simulink model "fangbo_pll_eso_J_identification"  (R2018b)
settings: Solver=FixedStepAuto  StartTime=0.0  StopTime=0.2  FixedStep=1e-7  RelTol=1e-3
InitFcn:
  | Vin1=30;%注入高频信号幅值
  | fin1=5000;%注入高频信号频率
  | fpwm=10000;%电流环控制频率
  | Tpwm=1/fpwm;
  | Tspd=Tpwm*10;%速度环控制周期（未用）
  | Td=2e-6;%逆变器死区时间（未加入）
  | Udc=90;
  | Pn=4;%极对数
  | R=0.281;
  | Ld=2.523e-3;Lq=5e-3;
  | faif=0.13455;
  | J=0.0012145+ 0.00126+0.0002601;%两个电机加联轴器
  | B=0.0006;
  | TL=10;%额定负载
  | nref=2200;%给定转速
  | %%%%%%luenberger观测器参数%%%%%%%
  | p=2*pi*10;%2;%极点位置，可调
  | eta=1;%1e-2;
  | alpha1=3*p;
  | alpha2=3*p^2;
  | alpha3=p^3;
  | %%%%%%锁相环参数%%%%%%%%%%%%%%%%%
  | Kppll= 300;   %2*p
  | Kipll= 1000;  %p^2
  | %%%%%%%%%双闭环3对PI参数%%%%%%%%%
  | BWc=300*2*pi;%电流环带宽
  | h=6;%速度环中频宽
  | K1=9.55*1.5*Pn*faif/J;
  | wcon=200*2*pi;%转速环反馈滤波和给定滤波器截止频率
  | Tsn=1/BWc+1/wcon;
  | Kpd=BWc*Ld;
  | Kid=R/Ld;
  | Kpq=BWc*Lq;
  | Kiq=R/Lq;
  | Kps=(h+1)/(2*h*Tsn*K1);
  | Kis=1/(h*Tsn);
  | %BWs=15*2*pi;
  | %Kps=BWs/K1;
  | %Kis=Kps*BWs/5;
  | %%%%%%%%%%%扰动观测器PID参数%%%%%%%%%%%%%
  | pd=2*pi*50;
  | kd_d=3*pd;
  | kp_d=3*pd^2;
  | ki_d=pd^3;
undefined symbols (not defined in the file): DiscIntNeverNeededParam, fin
libraries: simulink x16, dsparch4 x7, powerlib x5, dspsrcs4 x2, powerlib_meascontrol x2
(part 1 of 2)
settings Model: Creator=TAH  LastModifiedBy=Think
settings DebuggingCC: LibraryContextMissingDiagnostic=none
settings SFSimCC: SimUseLocalCustomCode=off
settings RTWCC: RTWUseLocalCustomCode=off
settings CodeAppCC: StateflowObjectComments=on
settings SimscapeCC: SimscapeNormalizeSystem=off

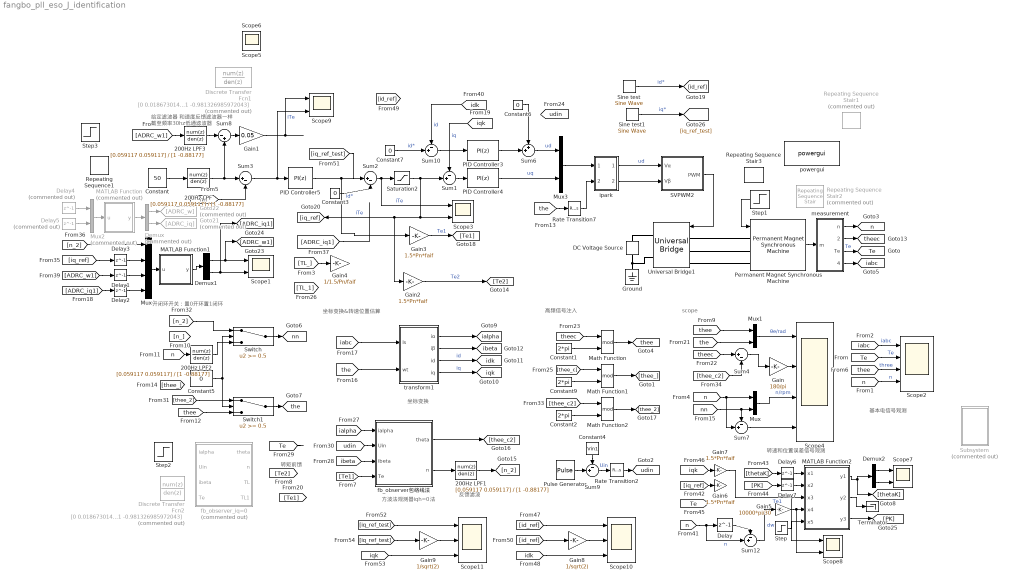
== system fangbo_pll_eso_J_identification ==
  note: 基本电信号观测
  note: 转速和位置误差信号观测
  note: 坐标变换
  note: 给定滤波器
      | 和速度反馈滤波器一样
      | 截至频率30hz低通滤波器
  note: 开闭环开关：置0开环置1闭环
  note: 坐标变换&转速位置估算
  note: 高频信号注入
  note: scope
  note: 方波法观测器iqh=0法
  note: 转矩前馈
  note: 反馈滤波
  200Hz LPF{,1..3} (4 alike) : DiscreteTransferFcn  Numerator=[0.059117 0.059117]  Denominator=[1 -0.88177]  SampleTime=Tpwm
  Constant : Constant  Value=50
  Constant1 : Constant  Value=2*pi  SampleTime=Tpwm
  Constant2 : Constant  Value=2*pi  SampleTime=Tpwm
  Constant3 : Constant  Value=0  SampleTime=1e-4
  Constant4 : Constant  Value=Vin1
  Constant5 : Constant  Value=0
  Constant6 : Constant  Value=0  SampleTime=1e-4
  Constant7 : Constant  Value=0  SampleTime=1e-4
  Constant9 : Constant  Value=2*pi  SampleTime=Tpwm
  DC Voltage Source : powerlib/Electrical Sources/DC Voltage Source  Amplitude=Udc  Measurements=None
      settings: SourceProductName=Simscape Electrical
  Delay{,1..3,6..7} (6 alike) : Delay  DelayLength=1  InitialCondition=0  UseCircularBuffer=on
  Delay4 : Delay  Commented=on  DelayLength=1  InitialCondition=0  UseCircularBuffer=on
  Delay5 : Delay  Commented=on  DelayLength=1  InitialCondition=0  UseCircularBuffer=on
  Demux : Demux  Commented=on  Outputs=2
  Demux1 : Demux  Outputs=2
  Demux2 : Demux  Outputs=2
  Discrete Transfer Fcn1 : DiscreteTransferFcn  Commented=on  Numerator=[0 0.018673014027957]  Denominator=[1 -0.981326985972043]  SampleTime=Tpwm
  Discrete Transfer Fcn2 : DiscreteTransferFcn  Commented=on  Numerator=[0 0.018673014027957]  Denominator=[1 -0.981326985972043]  SampleTime=Tpwm
  Gain : Gain  Gain=180/pi
  Gain1 : Gain  Gain=0.05
  Gain{2..3,6..7} (4 alike) : Gain  Gain=1.5*Pn*faif
  Gain4 : Gain  Gain=1/1.5/Pn/faif
  Gain5 : Gain  Gain=10000*pi/30
  Gain8 : Gain  Gain=1/sqrt(2)
  Gain9 : Gain  Gain=1/sqrt(2)
  Goto21 : Goto  Commented=on  GotoTag=ADRC_iq
  Goto22 : Goto  Commented=on  GotoTag=ADRC_w
  Ground : powerlib/Elements/Ground  LConnTagsString=a
      settings: SourceProductName=Simscape Electrical
  MATLAB Function : MATLAB Function  Commented=on  TreatAsAtomicUnit=on
  MATLAB Function1 : MATLAB Function  TreatAsAtomicUnit=on
  MATLAB Function2 : MATLAB Function  TreatAsAtomicUnit=on
  Math Function : Math  Operator=mod  SaturateOnIntegerOverflow=on
  Math Function1 : Math  Operator=mod  SaturateOnIntegerOverflow=on
  Math Function2 : Math  Operator=mod  SaturateOnIntegerOverflow=on
  Mux : Mux  Inputs=2
  Mux1 : Mux  Inputs=2
  Mux2 : Mux  Commented=on  Inputs=2
  Mux3 : Mux  Inputs=2
  Mux4 : Mux
  PID Controller3 : simulink/Continuous/PID Controller  Controller=PI  Form=Ideal  TimeDomain=Discrete-time  SampleTime=Tpwm  IntegratorMethod=Forward Euler  FilterMethod=Forward Euler  ControllerParametersSource=internal  P=Kpd  I=Kid  D=0  UseFilter=on  N=100  TunerSelectOption=Transfer Function Based (PID Tuner App)  InitialConditionSource=internal  InitialConditionForIntegrator=0  InitialConditionForFilter=0  DifferentiatorICPrevScaledInput=0  ExternalReset=none  TrackingMode=off  Kt=1  LimitOutput=on  UpperSaturationLimit=Udc/sqrt(3)  LowerSaturationLimit=-Udc/sqrt(3)  LinearizeAsGain=on  AntiWindupMode=none  Kb=1  POutMin=[]  POutMax=[]  IOutMin=[]  IOutMax=[]  DOutMin=[]  DOutMax=[]  NOutMin=[]  NOutMax=[]  SumOutMin=[]  SumOutMax=[]  SaturationOutMin=[]  SaturationOutMax=[]  PParamMin=[]  PParamMax=[]  IParamMin=[]  IParamMax=[]  DParamMin=[]  DParamMax=[]  NParamMin=[]  NParamMax=[]  KbParamMin=[]  KbParamMax=[]  KtParamMin=[]  KtParamMax=[]  KbOutMin=[]  KbOutMax=[]  KtOutMin=[]  KtOutMax=[]  IntegratorOutMin=[]  IntegratorOutMax=[]  FilterOutMin=[]  FilterOutMax=[]  SumI1OutMin=[]  SumI1OutMax=[]  SumI2OutMin=[]  SumI2OutMax=[]  SumI3OutMin=[]  SumI3OutMax=[]  SumI4OutMin=[]  SumI4OutMax=[]  SumDOutMin=[]  SumDOutMax=[]  DifferentiatorOutMin=[]  DifferentiatorOutMax=[]  FilterDiffOutCoefMin=[]  FilterDiffOutCoefMax=[]  ReciprocalOutMin=[]  ReciprocalOutMax=[]  SumDenOutMin=[]  SumDenOutMax=[]  SumNumOutMin=[]  SumNumOutMax=[]  DivideOutMin=[]  DivideOutMax=[]  IntegratorContinuousStateAttributes=''  IntegratorStateMustResolveToSignalObject=off  IntegratorRTWStateStorageClass=Auto  FilterContinuousStateAttributes=''  FilterStateMustResolveToSignalObject=off  FilterRTWStateStorageClass=Auto  ParallelPVariant=Passthrough  IdealPVariant=InternalParameters  IVariant=InternalParameters  DVariant=Disabled  IntegratorVariant=Discrete  SatVariant=Enabled  AWVariant=Passthrough  PCopyVariant=Disabled  TRVariant=Disabled  FdbkBlocksVariant=Forward  IdealPFdbkVariant=Disabled  SatFdbkVariant=Disabled  DerivativeFilterVariant=Disabled  NVariant=Disabled  NCopyVariant=Disabled_SignalSpec  FilterICVariant=Disabled  IntegratorICVariant=InternalICs  ExternalResetVariant=Disabled  TRSumVariant=Passthrough  SumFdbkVariant=Disabled  SumVariant=Sum_PI
  PID Controller4 : simulink/Continuous/PID Controller  Controller=PI  Form=Ideal  TimeDomain=Discrete-time  SampleTime=Tpwm  IntegratorMethod=Forward Euler  FilterMethod=Forward Euler  ControllerParametersSource=internal  P=Kpq  I=Kiq  D=0  UseFilter=on  N=100  TunerSelectOption=Transfer Function Based (PID Tuner App)  InitialConditionSource=internal  InitialConditionForIntegrator=0  InitialConditionForFilter=0  DifferentiatorICPrevScaledInput=0  ExternalReset=none  TrackingMode=off  Kt=1  LimitOutput=on  UpperSaturationLimit=Udc/sqrt(3)  LowerSaturationLimit=-Udc/sqrt(3)  LinearizeAsGain=on  AntiWindupMode=none  Kb=1  POutMin=[]  POutMax=[]  IOutMin=[]  IOutMax=[]  DOutMin=[]  DOutMax=[]  NOutMin=[]  NOutMax=[]  SumOutMin=[]  SumOutMax=[]  SaturationOutMin=[]  SaturationOutMax=[]  PParamMin=[]  PParamMax=[]  IParamMin=[]  IParamMax=[]  DParamMin=[]  DParamMax=[]  NParamMin=[]  NParamMax=[]  KbParamMin=[]  KbParamMax=[]  KtParamMin=[]  KtParamMax=[]  KbOutMin=[]  KbOutMax=[]  KtOutMin=[]  KtOutMax=[]  IntegratorOutMin=[]  IntegratorOutMax=[]  FilterOutMin=[]  FilterOutMax=[]  SumI1OutMin=[]  SumI1OutMax=[]  SumI2OutMin=[]  SumI2OutMax=[]  SumI3OutMin=[]  SumI3OutMax=[]  SumI4OutMin=[]  SumI4OutMax=[]  SumDOutMin=[]  SumDOutMax=[]  DifferentiatorOutMin=[]  DifferentiatorOutMax=[]  FilterDiffOutCoefMin=[]  FilterDiffOutCoefMax=[]  ReciprocalOutMin=[]  ReciprocalOutMax=[]  SumDenOutMin=[]  SumDenOutMax=[]  SumNumOutMin=[]  SumNumOutMax=[]  DivideOutMin=[]  DivideOutMax=[]  IntegratorContinuousStateAttributes=''  IntegratorStateMustResolveToSignalObject=off  IntegratorRTWStateStorageClass=Auto  FilterContinuousStateAttributes=''  FilterStateMustResolveToSignalObject=off  FilterRTWStateStorageClass=Auto  ParallelPVariant=Passthrough  IdealPVariant=InternalParameters  IVariant=InternalParameters  DVariant=Disabled  IntegratorVariant=Discrete  SatVariant=Enabled  AWVariant=Passthrough  PCopyVariant=Disabled  TRVariant=Disabled  FdbkBlocksVariant=Forward  IdealPFdbkVariant=Disabled  SatFdbkVariant=Disabled  DerivativeFilterVariant=Disabled  NVariant=Disabled  NCopyVariant=Disabled_SignalSpec  FilterICVariant=Disabled  IntegratorICVariant=InternalICs  ExternalResetVariant=Disabled  TRSumVariant=Passthrough  SumFdbkVariant=Disabled  SumVariant=Sum_PI
  PID Controller5 : simulink/Continuous/PID Controller  Controller=PI  Form=Ideal  TimeDomain=Discrete-time  SampleTime=Tpwm  IntegratorMethod=Forward Euler  FilterMethod=Forward Euler  ControllerParametersSource=internal  P=Kps  I=Kis  D=0  UseFilter=on  N=100  TunerSelectOption=Transfer Function Based (PID Tuner App)  InitialConditionSource=internal  InitialConditionForIntegrator=0  InitialConditionForFilter=0  DifferentiatorICPrevScaledInput=0  ExternalReset=none  TrackingMode=off  Kt=1  LimitOutput=on  UpperSaturationLimit=15  LowerSaturationLimit=-15  LinearizeAsGain=on  AntiWindupMode=none  Kb=1  POutMin=[]  POutMax=[]  IOutMin=[]  IOutMax=[]  DOutMin=[]  DOutMax=[]  NOutMin=[]  NOutMax=[]  SumOutMin=[]  SumOutMax=[]  SaturationOutMin=[]  SaturationOutMax=[]  PParamMin=[]  PParamMax=[]  IParamMin=[]  IParamMax=[]  DParamMin=[]  DParamMax=[]  NParamMin=[]  NParamMax=[]  KbParamMin=[]  KbParamMax=[]  KtParamMin=[]  KtParamMax=[]  KbOutMin=[]  KbOutMax=[]  KtOutMin=[]  KtOutMax=[]  IntegratorOutMin=[]  IntegratorOutMax=[]  FilterOutMin=[]  FilterOutMax=[]  SumI1OutMin=[]  SumI1OutMax=[]  SumI2OutMin=[]  SumI2OutMax=[]  SumI3OutMin=[]  SumI3OutMax=[]  SumI4OutMin=[]  SumI4OutMax=[]  SumDOutMin=[]  SumDOutMax=[]  DifferentiatorOutMin=[]  DifferentiatorOutMax=[]  FilterDiffOutCoefMin=[]  FilterDiffOutCoefMax=[]  ReciprocalOutMin=[]  ReciprocalOutMax=[]  SumDenOutMin=[]  SumDenOutMax=[]  SumNumOutMin=[]  SumNumOutMax=[]  DivideOutMin=[]  DivideOutMax=[]  IntegratorContinuousStateAttributes=''  IntegratorStateMustResolveToSignalObject=off  IntegratorRTWStateStorageClass=Auto  FilterContinuousStateAttributes=''  FilterStateMustResolveToSignalObject=off  FilterRTWStateStorageClass=Auto  ParallelPVariant=Passthrough  IdealPVariant=InternalParameters  IVariant=InternalParameters  DVariant=Disabled  IntegratorVariant=Discrete  SatVariant=Enabled  AWVariant=Passthrough  PCopyVariant=Disabled  TRVariant=Disabled  FdbkBlocksVariant=Forward  IdealPFdbkVariant=Disabled  SatFdbkVariant=Disabled  DerivativeFilterVariant=Disabled  NVariant=Disabled  NCopyVariant=Disabled_SignalSpec  FilterICVariant=Disabled  IntegratorICVariant=InternalICs  ExternalResetVariant=Disabled  TRSumVariant=Passthrough  SumFdbkVariant=Disabled  SumVariant=Sum_PI
  Permanent Magnet Synchronous Machine : powerlib/Machines/Permanent Magnet Synchronous Machine  NbPhases=3  FluxDistribution=Sinusoidal  RotorType=Salient-pole  MechanicalLoad=Torque Tm  PresetModel=No  ShowDetailedParameters=on  MeasurementBus=off  Resistance=R  Inductance=8.5e-3  dqInductances=[Ld Lq]  La=0.000395  MachineConstant=Flux linkage established by magnets (V.s)  Flux=faif  VoltageCst=97.6187  TorqueCst=0.8073  Flat=120  Mechanical=[J 0 Pn 0]  PolePairs=2  InitialConditions=[0,0, 0,0]  InitialConditions5ph=[0 0 0 0 0 0]  TsPowergui=0  TsBlock=-1  RefAngle=Aligned with phase A axis (original Park)
  Pulse Generator : DiscretePulseGenerator  PulseType=Time based  Amplitude=2*Vin1  Period=2*Tpwm  PulseWidth=50  VectorParams1D=off
  Rate Transition2 : RateTransition  OutPortSampleTime=1e-4
  Rate Transition7 : RateTransition  OutPortSampleTime=Tpwm
  Repeating Sequence Stair1 : simulink/Sources/Repeating Sequence Stair  Commented=on  OutValues=[0 5 0 ].'  tsamp=0.2  OutMin=[]  OutMax=[]  OutDataTypeStr=double  OutputDataTypeScalingMode=double  OutDataType=fixdt(0,8)  ConRadixGroup=Best Precision: Vector-wise  OutScaling=2^-12
  Repeating Sequence Stair2 : simulink/Sources/Repeating Sequence Stair  Commented=on  OutValues=[0 0.5*TL 0.5*TL 0.5*TL 0.5*TL].'  tsamp=0.2  OutMin=[]  OutMax=[]  OutDataTypeStr=double  OutputDataTypeScalingMode=double  OutDataType=fixdt(0,8)  ConRadixGroup=Best Precision: Vector-wise  OutScaling=2^-12
  Repeating Sequence Stair3 : simulink/Sources/Repeating Sequence Stair  OutValues=[2 2 2 ].'  tsamp=0.2  OutMin=[]  OutMax=[]  OutDataTypeStr=double  OutputDataTypeScalingMode=double  OutDataType=fixdt(0,8)  ConRadixGroup=Best Precision: Vector-wise  OutScaling=2^-12
  Repeating Sequence1 : simulink/Sources/Repeating Sequence  rep_seq_t=[0 0.2 0.4 0.6]  rep_seq_y=[0 50 100 150]
  SVPWM2 : Subsystem
  Saturation2 : Saturate  UpperLimit=15  LowerLimit=-15
  Scope{1,3,7..9} (5 alike) : Scope  NumInputPorts=2
  Scope10 : Scope  NumInputPorts=3
  Scope11 : Scope  NumInputPorts=3
  Scope2 : Scope  NumInputPorts=4
  Scope4 : Scope  NumInputPorts=4
  Sine test : dspsrcs4/Sine Wave  Amplitude=5  Frequency=300  Phase=0  SampleMode=Discrete  OutComplex=Real  CompMethod=Trigonometric fcn  TableSize=Speed  SampleTime=1e-4  SamplesPerFrame=1  ResetState=Restart at time zero  OutputFrames=off  dataType=double  wordLen=16  udDataType=sfix(16)  fracBitsMode=Best precision  numFracBits=15  OutDataTypeStr=double  LastOutDataTypeStr=double
  Sine test1 : dspsrcs4/Sine Wave  Amplitude=5  Frequency=300  Phase=0  SampleMode=Discrete  OutComplex=Real  CompMethod=Trigonometric fcn  TableSize=Speed  SampleTime=1e-4  SamplesPerFrame=1  ResetState=Restart at time zero  OutputFrames=off  dataType=double  wordLen=16  udDataType=sfix(16)  fracBitsMode=Best precision  numFracBits=15  OutDataTypeStr=double  LastOutDataTypeStr=double
  Step : Step  Time=0.1  SampleTime=1e-4
  Step1 : Step  Time=0.2  After=0  SampleTime=1e-4
  Step2 : Step  Time=0.2  After=2  SampleTime=1e-4  VectorParams1D=off
  Step3 : Step  Time=0.1  Before=200  After=500  SampleTime=0
  Subsystem : Subsystem  Commented=on
  Sum{1,7,9..10,12} (5 alike) : Sum  Inputs=-+|
  Sum2 : Sum  Inputs=|+-
  Sum3 : Sum  Inputs=|+-
  Sum4 : Sum  Inputs=|+-
  Sum6 : Sum  Inputs=++|
  Sum8 : Sum  Inputs=|-+
  Switch : Switch  Threshold=0.5
  Switch1 : Switch  Threshold=0.5
  Terminator : Terminator
  Universal Bridge1 : powerlib/Power Electronics/Universal Bridge  Arms=3  SnubberResistance=1e5  SnubberCapacitance=inf  Device=IGBT / Diodes  Ron=1e-3  Lon=0  ForwardVoltages="[  0  0  ]"  ForwardVoltage=0  GTOparameters=[ 10e-6 , 20e-6 ]  IGBTparameters=[ 1e-6 , 2e-6 ]  Measurements=None  Measurements_2=None  converterType=Rectifier
      settings: SourceProductName=Simscape Electrical
  fb_observer_iq=0 : Subsystem  Commented=on
  fb_observer包络线法 : Subsystem
  ipark : Subsystem
      mask Display:
      | plot([0 1], [0,1])
      | port_label('input', 1, 'dq')
      | port_label('input', 2, 'wt')
      | port_label('output', 1, '\alpha\beta','texmode','on')
  measurement : Subsystem
  powergui : powerlib/powergui  Priority=1  SimulationMode=Discrete  SampleTime=1e-7  frequency=60  Iterations=50  frequencyindice=0  Pbase=100e6  ErrMax=1e-4  UnitsV=kV  UnitsW=MW  buscounter=0  FunctionMessages=off  echomessages=off  EnableUseOfTLC=off  CurrentSourceSwitches=off  DisableSnubberDevices=off  DisableRonSwitches=off  DisableVfSwitches=off  DisplayEquations=off  SolverType=Tustin/Backward Euler (TBE)  Interpol=off  ExternalGateDelay=off  methode=off  Ts=100  x0status=blocks  SPID=off  SwTol=0  HookPort=off  RestoreLinks=warning  ResistiveCurrentMeasurement=off  Frange=[0:2:500]  Ylog=off  Xlog=on  ShowGrid=off  save=off  variable=ZData  structure=test  ZoomFFT=off  StartTime=0.18  cycles=1  DisplayStyle=1  fundamental=3.333333333333333333  FreqAxis=off  MaxFrequency=1020  frequencyindicesteady=1  RmsSteady=1  display=off
  transform1 : Subsystem
  Scope5 : Scope
  Scope6 : Scope
  tag scope: Te=global, iabc=global, ialpha=global, ibeta=global, idk=global, iqk=global, n=global, nn=global, the=global, thee=global, theec=global, udin=global
  wires:
  Permanent Magnet Synchronous Machine/1 -> measurement/1(m)
  measurement/3(Te) -> [Te]  "Te"
  measurement/1(n) -> [n]
  measurement/4(iabc) -> [iabc]
  ipark/1(alpha) -> SVPWM2/1(Vα)  "ud"
  ipark/2(beta) -> SVPWM2/2(Vβ)
  Mux3/1 -> ipark/1(dq)
  Rate Transition7/1 -> ipark/2(wt)
  Sum6/1 -> Mux3/1  "ud"
  [iabc] -> Scope2/1  "iabc"
  [Te] -> Scope2/2  "Te"
  [n] -> Scope2/4  "n"
  [thee] -> Scope2/3  "three"
  Sum1/1 -> PID Controller4/1
  Sum3/1 -> PID Controller5/1, Scope9/2
  Sum10/1 -> PID Controller3/1
  [n_2] -> Switch/1
  [thee_2] -> Switch1/1
  Switch/1 -> [nn]
  Switch1/1 -> [the]
  Constant5/1 -> Switch/2, Switch1/2
  [thee] -> Switch1/3
  [n] -> Sum7/2, Mux/1
  Mux/1 -> Scope4/3  "n/rpm"
  Mux1/1 -> Scope4/1  "θe/rad"
  [thee] -> Mux1/1
  [the] -> Mux1/2
  [nn] -> Sum7/1, Mux/2
  transform1/3(id) -> [idk]  "id"
  transform1/4(iq) -> [iqk]  "iq"
  Constant9/1 -> Math Function1/2
  Math Function1/1 -> [thee_]
  [iabc] -> transform1/1(Is)
  [the] -> transform1/2(wt)
  [the] -> Rate Transition7/1
  [n] -> 200Hz LPF2/1
  200Hz LPF2/1 -> Switch/3
  200Hz LPF/1 -> Sum3/1, Sum8/2
  SVPWM2/1(PWM) -> Universal Bridge1/1
  Sum7/1 -> Scope4/4
  Constant1/1 -> Math Function/2
  measurement/2(thee) -> [theec]
  Math Function/1 -> [thee]
  [theec] -> Sum4/1
  [theec] -> Math Function/1
  PID Controller3/1 -> Sum6/2
  Constant6/1 -> Sum6/1
  [thee_c] -> Math Function1/1
  [iqk] -> Sum1/1  "iq"
  PID Controller4/1 -> Mux3/2  "uq"
  Pulse Generator/1 -> Sum9/2
  Constant4/1 -> Sum9/1
  Rate Transition2/1 -> [udin]
  Sum9/1 -> Rate Transition2/1  "Uin"
  [Te] -> ?
  [udin] -> fb_observer包络线法/2(Uin)
  [ialpha] -> fb_observer包络线法/1(ialpha)
  fb_observer包络线法/1(theta) -> [thee_c2]
  [thee_c2] -> Math Function2/1
  Math Function2/1 -> [thee_2]
  Constant2/1 -> Math Function2/2
  [thee_c2] -> Sum4/2
  Constant7/1 -> Sum10/2  "id*"
  Gain/1 -> Scope4/2
  Sum4/1 -> Gain/1
  Gain1/1 -> Scope9/1  "iTe"
  Gain2/1 -> [Te2]  "Te2"
  Gain3/1 -> [Te1]  "Te1"
  transform1/1(iα) -> [ialpha]
  transform1/2(iβ) -> [ibeta]
  [ibeta] -> fb_observer包络线法/3(ibeta)
  Step1/1 -> Permanent Magnet Synchronous Machine/1
  [Te1] -> fb_observer包络线法/4(Te)
  [TL_] -> Gain4/1
  Mux2/1 -> MATLAB Function/1(u)
  MATLAB Function/1(y) -> Demux/1
  Demux/2 -> Goto21/1
  Sum8/1 -> Gain1/1
  fb_observer包络线法/2(n) -> 200Hz LPF1/1
  200Hz LPF1/1 -> [n_2]
  [n_2] -> Mux4/1
  [iq_ref] -> Delay3/1
  [nn] -> Sum3/2
  Delay4/1 -> Mux2/1
  Delay3/1 -> Mux4/2
  [ADRC_w1] -> 200Hz LPF3/1
  [idk] -> Sum10/1  "id"
  200Hz LPF3/1 -> Sum8/1
  Sum2/1 -> Scope3/1, Saturation2/1  "iTe"
  Demux/1 -> Goto22/1
  [ADRC_iq1] -> Delay2/1
  Delay2/1 -> Mux4/4
  Delay1/1 -> Mux4/3
  [ADRC_w1] -> Delay1/1
  Saturation2/1 -> Sum1/2, Scope3/2, [iq_ref], Gain2/1  "iTe"
  Mux4/1 -> MATLAB Function1/1(u)
  MATLAB Function1/1(y) -> Demux1/1
  Demux1/1 -> [ADRC_w1], Scope1/1
  Demux1/2 -> [ADRC_iq1], Scope1/2
  [ADRC_iq1] -> ?
  Delay5/1 -> Mux2/2
  PID Controller5/1 -> Gain3/1
  [n] -> Sum12/2, Delay/1  "n"
  Delay/1 -> Sum12/1
  Sum12/1 -> Gain5/1  "dw"
  Gain5/1 -> Scope8/2, MATLAB Function2/4(x4)
  Gain7/1 -> Scope8/1, MATLAB Function2/3(x3)  "Te1"
  [iq_ref] -> Gain6/1
  MATLAB Function2/1(y1) -> [thetaK], Demux2/1
  MATLAB Function2/2(y2) -> Terminator/1
  MATLAB Function2/3(y3) -> [PK]
  [thetaK] -> Delay6/1
  Delay6/1 -> MATLAB Function2/1(x1)
  Delay7/1 -> MATLAB Function2/2(x2)
  [PK] -> Delay7/1
  Demux2/1 -> Scope7/1
  Demux2/2 -> Scope7/2
  Step/1 -> MATLAB Function2/5(x5)
  [iqk] -> Gain7/1
  Constant/1 -> 200Hz LPF/1
  Constant3/1 -> Sum2/2  "id*"
  Sine test/1 -> [id_ref]  "id*"
  [id_ref] -> Scope10/1
  [idk] -> Scope10/3
  [id_ref] -> Gain8/1
  Gain8/1 -> Scope10/2
  Sine test1/1 -> [iq_ref_test]  "iq*"
  [iq_ref_test] -> Sum2/1
  Gain9/1 -> Scope11/2
  [iq_ref_test] -> Gain9/1
  [iqk] -> Scope11/3
  [iq_ref_test] -> Scope11/1
  connections:
  DC Voltage Source/LConn1 -- Universal Bridge1/RConn2 -- Ground/LConn1
  Universal Bridge1/LConn2 -- Permanent Magnet Synchronous Machine/LConn2
  Universal Bridge1/LConn3 -- Permanent Magnet Synchronous Machine/LConn3
  Universal Bridge1/RConn1 -- DC Voltage Source/RConn1
  Universal Bridge1/LConn1 -- Permanent Magnet Synchronous Machine/LConn1

== system fangbo_pll_eso_J_identification/SVPWM2 ==
  Vα : Inport
  Vβ : Inport  Port=2
  CMP3 : Subsystem
  PWMlixiang : Subsystem
  PWMsiqu1 : Subsystem  Commented=on
  Scope1 : Scope
  TxTy : Subsystem
  sector : Subsystem
  PWM : Outport
  wires:
  Vα/1 -> sector/1(Ualpha), TxTy/1(Vsalpha)
  Vβ/1 -> sector/2(Ubeta), TxTy/2(Vsbelta)
  sector/1(sector) -> Scope1/1, CMP3/1(sector), TxTy/3(sector)
  TxTy/1(Tx) -> CMP3/2(tx)
  TxTy/2(Ty) -> CMP3/3(ty)
  CMP3/2(CMPB) -> PWMsiqu1/2(CMP2), PWMlixiang/2(CMP2)
  CMP3/3(CMPC) -> PWMsiqu1/3(CMP3), PWMlixiang/3(CMP3)
  CMP3/1(CMPA) -> PWMlixiang/1(CMP1), PWMsiqu1/1(CMP1)
  PWMlixiang/1(PWM) -> PWM/1

== system fangbo_pll_eso_J_identification/Subsystem ==
  note: 反馈滤波
  note: 转矩前馈
  note: 方波法观测器包络线法
  Discrete Transfer Fcn2 : DiscreteTransferFcn  Commented=on  Numerator=[0 0.018673014027957]  Denominator=[1 -0.981326985972043]  SampleTime=Tpwm
  From15 : From  Commented=on  GotoTag=ialpha  TagVisibility=global
  From21 : From  Commented=on  GotoTag=ibeta  TagVisibility=global
  From26 : From  Commented=on  GotoTag=Te  TagVisibility=global
  From3 : From  Commented=on  GotoTag=udin  TagVisibility=global
  Goto14 : Goto  Commented=on  GotoTag=n_
  Goto8 : Goto  Commented=on  GotoTag=thee_c
  fb_observer : Subsystem  Commented=on
  wires:
  Discrete Transfer Fcn2/1 -> Goto14/1
  fb_observer/1(theta) -> Goto8/1
  fb_observer/2(n) -> Discrete Transfer Fcn2/1
  From15/1 -> fb_observer/1(ialpha)
  From21/1 -> fb_observer/3(ibeta)
  From3/1 -> fb_observer/2(Uin)
  From26/1 -> fb_observer/4(Te)

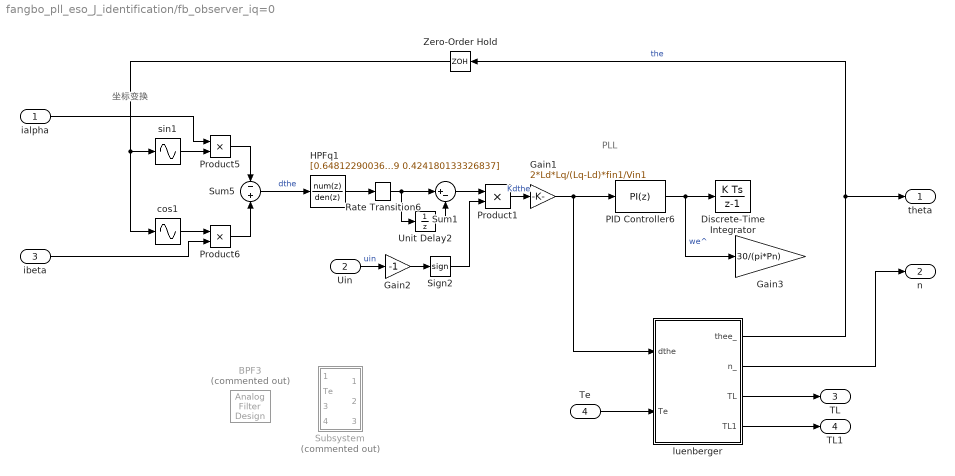
== system fangbo_pll_eso_J_identification/fb_observer_iq=0 ==
  note: 坐标变换
  note: PLL
  ialpha : Inport
  Uin : Inport  Port=2
  ibeta : Inport  Port=3
  Te : Inport  Port=4
  BPF3 : dsparch4/Analog Filter Design  Commented=on  method=Butterworth  filttype=Highpass  N=1  Wlo=500*2*pi  Whi=(fin+200)*2*pi  Rp=2  Rs=40
  Discrete-Time Integrator : DiscreteIntegrator  SampleTime=Tpwm  ICPrevOutput=DiscIntNeverNeededParam  ICPrevScaledInput=DiscIntNeverNeededParam
  Gain1 : Gain  Gain=2*Ld*Lq/(Lq-Ld)*fin1/Vin1
  Gain2 : Gain  Gain=-1
  Gain3 : Gain  Gain=30/(pi*Pn)
  HPFq1 : DiscreteTransferFcn  Numerator=[0.648122900364569 -1.296245800729138 0.648122900364569]  Denominator=[1 -1.168311468131439 0.424180133326837]  SampleTime=Tpwm
  PID Controller6 : simulink/Continuous/PID Controller  Controller=PI  Form=Parallel  TimeDomain=Discrete-time  SampleTime=Tpwm  IntegratorMethod=Forward Euler  FilterMethod=Forward Euler  ControllerParametersSource=internal  P=Kppll  I=Kipll  D=0  UseFilter=on  N=100  TunerSelectOption=Transfer Function Based (PID Tuner App)  InitialConditionSource=internal  InitialConditionForIntegrator=0  InitialConditionForFilter=0  DifferentiatorICPrevScaledInput=0  ExternalReset=none  TrackingMode=off  Kt=1  LimitOutput=off  UpperSaturationLimit=inf  LowerSaturationLimit=-inf  LinearizeAsGain=on  AntiWindupMode=none  Kb=1  POutMin=[]  POutMax=[]  IOutMin=[]  IOutMax=[]  DOutMin=[]  DOutMax=[]  NOutMin=[]  NOutMax=[]  SumOutMin=[]  SumOutMax=[]  SaturationOutMin=[]  SaturationOutMax=[]  PParamMin=[]  PParamMax=[]  IParamMin=[]  IParamMax=[]  DParamMin=[]  DParamMax=[]  NParamMin=[]  NParamMax=[]  KbParamMin=[]  KbParamMax=[]  KtParamMin=[]  KtParamMax=[]  KbOutMin=[]  KbOutMax=[]  KtOutMin=[]  KtOutMax=[]  IntegratorOutMin=[]  IntegratorOutMax=[]  FilterOutMin=[]  FilterOutMax=[]  SumI1OutMin=[]  SumI1OutMax=[]  SumI2OutMin=[]  SumI2OutMax=[]  SumI3OutMin=[]  SumI3OutMax=[]  SumI4OutMin=[]  SumI4OutMax=[]  SumDOutMin=[]  SumDOutMax=[]  DifferentiatorOutMin=[]  DifferentiatorOutMax=[]  FilterDiffOutCoefMin=[]  FilterDiffOutCoefMax=[]  ReciprocalOutMin=[]  ReciprocalOutMax=[]  SumDenOutMin=[]  SumDenOutMax=[]  SumNumOutMin=[]  SumNumOutMax=[]  DivideOutMin=[]  DivideOutMax=[]  IntegratorContinuousStateAttributes=''  IntegratorStateMustResolveToSignalObject=off  IntegratorRTWStateStorageClass=Auto  FilterContinuousStateAttributes=''  FilterStateMustResolveToSignalObject=off  FilterRTWStateStorageClass=Auto  ParallelPVariant=InternalParameters  IdealPVariant=Disabled  IVariant=InternalParameters  DVariant=Disabled  IntegratorVariant=Discrete  SatVariant=Disabled  AWVariant=Passthrough  PCopyVariant=Disabled  TRVariant=Disabled  FdbkBlocksVariant=Forward  IdealPFdbkVariant=Disabled  SatFdbkVariant=Disabled  DerivativeFilterVariant=Disabled  NVariant=Disabled  NCopyVariant=Disabled_SignalSpec  FilterICVariant=Disabled  IntegratorICVariant=InternalICs  ExternalResetVariant=Disabled  TRSumVariant=Passthrough  SumFdbkVariant=Disabled  SumVariant=Sum_PI
  Product1 : Product
  Product5 : Product
  Product6 : Product
  Rate Transition6 : RateTransition  OutPortSampleTime=Tpwm
  Sign2 : Signum
  Subsystem : Subsystem  Commented=on
  Sum1 : Sum  Inputs=|+-
  Sum5 : Sum  Inputs=-|+
  Unit Delay2 : UnitDelay  SampleTime=Tpwm
  Zero-Order Hold : ZeroOrderHold  SampleTime=Tpwm
  cos1 : Sin  TimeSource=Use external signal  Phase=pi/2  SampleTime=0
  luenberger : Subsystem
  sin1 : Sin  TimeSource=Use external signal  SampleTime=0
  theta : Outport
  n : Outport  Port=2
  TL : Outport  Port=3
  TL1 : Outport  Port=4
  wires:
  Uin/1 -> Gain2/1  "uin"
  Product5/1 -> Sum5/1
  luenberger/1(thee_) -> theta/1, Zero-Order Hold/1  "the"
  PID Controller6/1 -> Gain3/1, Discrete-Time Integrator/1  "we^"
  Sum5/1 -> HPFq1/1  "dthe"
  Product6/1 -> Sum5/2
  sin1/1 -> Product5/2
  cos1/1 -> Product6/1
  HPFq1/1 -> Rate Transition6/1
  Unit Delay2/1 -> Sum1/2
  Gain2/1 -> Sign2/1
  Product1/1 -> Gain1/1  "Kdthe"
  Sum1/1 -> Product1/1
  Sign2/1 -> Product1/2
  Te/1 -> luenberger/2(Te)
  luenberger/2(n_) -> n/1
  Gain1/1 -> luenberger/1(dthe), PID Controller6/1
  Rate Transition6/1 -> Unit Delay2/1, Sum1/1
  luenberger/3(TL) -> TL/1
  luenberger/4(TL1) -> TL1/1
  Zero-Order Hold/1 -> cos1/1, sin1/1
  ialpha/1 -> Product5/1
  ibeta/1 -> Product6/2

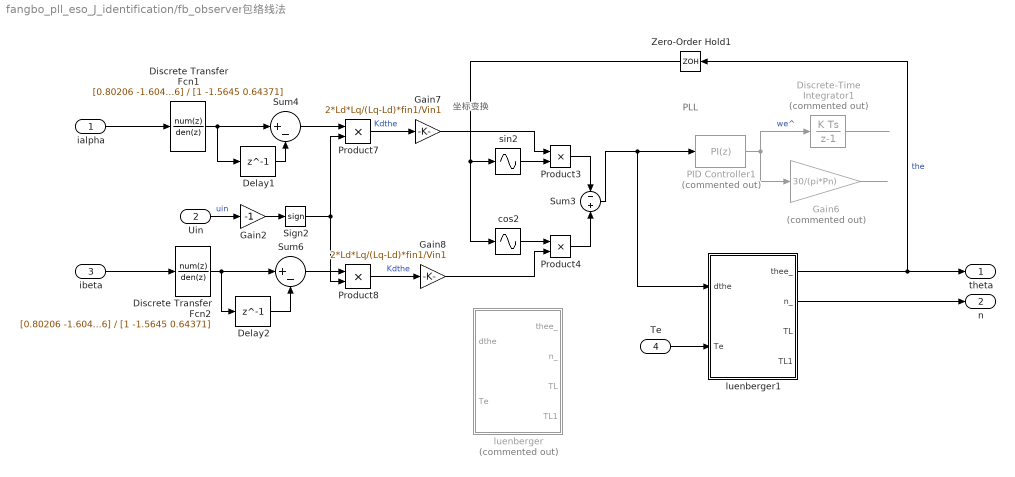
== system fangbo_pll_eso_J_identification/fb_observer包络线法 ==
  note: 坐标变换
  note: PLL
  ialpha : Inport
  Uin : Inport  Port=2
  ibeta : Inport  Port=3
  Te : Inport  Port=4
  Delay1 : Delay  DelayLength=1  SampleTime=Tpwm
  Delay2 : Delay  DelayLength=1  SampleTime=Tpwm
  Discrete Transfer Fcn1 : DiscreteTransferFcn  Numerator=[0.80206 -1.6041 0.80206]  Denominator=[1 -1.5645 0.64371]  SampleTime=Tpwm
  Discrete Transfer Fcn2 : DiscreteTransferFcn  Numerator=[0.80206 -1.6041 0.80206]  Denominator=[1 -1.5645 0.64371]  SampleTime=Tpwm
  Discrete-Time Integrator1 : DiscreteIntegrator  Commented=on  SampleTime=Tpwm  ICPrevOutput=DiscIntNeverNeededParam  ICPrevScaledInput=DiscIntNeverNeededParam
  Gain2 : Gain  Gain=-1
  Gain6 : Gain  Commented=on  Gain=30/(pi*Pn)
  Gain7 : Gain  Gain=2*Ld*Lq/(Lq-Ld)*fin1/Vin1
  Gain8 : Gain  Gain=2*Ld*Lq/(Lq-Ld)*fin1/Vin1
  PID Controller1 : simulink/Continuous/PID Controller  Commented=on  Controller=PI  Form=Parallel  TimeDomain=Discrete-time  SampleTime=Tpwm  IntegratorMethod=Forward Euler  FilterMethod=Forward Euler  ControllerParametersSource=internal  P=Kppll  I=Kipll  D=0  UseFilter=on  N=100  TunerSelectOption=Transfer Function Based (PID Tuner App)  InitialConditionSource=internal  InitialConditionForIntegrator=0  InitialConditionForFilter=0  DifferentiatorICPrevScaledInput=0  ExternalReset=none  TrackingMode=off  Kt=1  LimitOutput=off  UpperSaturationLimit=inf  LowerSaturationLimit=-inf  LinearizeAsGain=on  AntiWindupMode=none  Kb=1  POutMin=[]  POutMax=[]  IOutMin=[]  IOutMax=[]  DOutMin=[]  DOutMax=[]  NOutMin=[]  NOutMax=[]  SumOutMin=[]  SumOutMax=[]  SaturationOutMin=[]  SaturationOutMax=[]  PParamMin=[]  PParamMax=[]  IParamMin=[]  IParamMax=[]  DParamMin=[]  DParamMax=[]  NParamMin=[]  NParamMax=[]  KbParamMin=[]  KbParamMax=[]  KtParamMin=[]  KtParamMax=[]  KbOutMin=[]  KbOutMax=[]  KtOutMin=[]  KtOutMax=[]  IntegratorOutMin=[]  IntegratorOutMax=[]  FilterOutMin=[]  FilterOutMax=[]  SumI1OutMin=[]  SumI1OutMax=[]  SumI2OutMin=[]  SumI2OutMax=[]  SumI3OutMin=[]  SumI3OutMax=[]  SumI4OutMin=[]  SumI4OutMax=[]  SumDOutMin=[]  SumDOutMax=[]  DifferentiatorOutMin=[]  DifferentiatorOutMax=[]  FilterDiffOutCoefMin=[]  FilterDiffOutCoefMax=[]  ReciprocalOutMin=[]  ReciprocalOutMax=[]  SumDenOutMin=[]  SumDenOutMax=[]  SumNumOutMin=[]  SumNumOutMax=[]  DivideOutMin=[]  DivideOutMax=[]  IntegratorContinuousStateAttributes=''  IntegratorStateMustResolveToSignalObject=off  IntegratorRTWStateStorageClass=Auto  FilterContinuousStateAttributes=''  FilterStateMustResolveToSignalObject=off  FilterRTWStateStorageClass=Auto  ParallelPVariant=InternalParameters  IdealPVariant=Disabled  IVariant=InternalParameters  DVariant=Disabled  IntegratorVariant=Discrete  SatVariant=Disabled  AWVariant=Passthrough  PCopyVariant=Disabled  TRVariant=Disabled  FdbkBlocksVariant=Forward  IdealPFdbkVariant=Disabled  SatFdbkVariant=Disabled  DerivativeFilterVariant=Disabled  NVariant=Disabled  NCopyVariant=Disabled_SignalSpec  FilterICVariant=Disabled  IntegratorICVariant=InternalICs  ExternalResetVariant=Disabled  TRSumVariant=Passthrough  SumFdbkVariant=Disabled  SumVariant=Sum_PI
  Product{3..4,7..8} (4 alike) : Product
  Sign2 : Signum
  Sum3 : Sum  Inputs=-|+
  Sum4 : Sum  Inputs=|+-
  Sum6 : Sum  Inputs=|+-
  Zero-Order Hold1 : ZeroOrderHold  SampleTime=Tpwm
  cos2 : Sin  TimeSource=Use external signal  Phase=pi/2  SampleTime=0
  luenberger : Subsystem  Commented=on
  luenberger1 : Subsystem
  sin2 : Sin  TimeSource=Use external signal  SampleTime=0
  theta : Outport
  n : Outport  Port=2
  wires:
  Product4/1 -> Sum3/2
  sin2/1 -> Product3/2
  Zero-Order Hold1/1 -> cos2/1, sin2/1
  Gain7/1 -> Product3/1
  Gain8/1 -> Product4/2
  Gain6/1 -> ?
  ibeta/1 -> Discrete Transfer Fcn2/1
  Sum6/1 -> Product8/1
  Product7/1 -> Gain7/1  "Kdthe"
  Sign2/1 -> Product8/2, Product7/2
  cos2/1 -> Product4/1
  Sum4/1 -> Product7/1
  Uin/1 -> Gain2/1  "uin"
  Product8/1 -> Gain8/1  "Kdthe"
  Discrete-Time Integrator1/1 -> ?
  Gain2/1 -> Sign2/1
  Delay2/1 -> Sum6/2
  PID Controller1/1 -> Discrete-Time Integrator1/1, Gain6/1  "we^"
  Discrete Transfer Fcn1/1 -> Sum4/1, Delay1/1
  Discrete Transfer Fcn2/1 -> Sum6/1, Delay2/1
  Sum3/1 -> luenberger1/1(dthe), PID Controller1/1
  Product3/1 -> Sum3/1
  Te/1 -> luenberger1/2(Te)
  ialpha/1 -> Discrete Transfer Fcn1/1
  Delay1/1 -> Sum4/2
  luenberger1/1(thee_) -> Zero-Order Hold1/1, theta/1  "the"
  luenberger1/2(n_) -> n/1

== system fangbo_pll_eso_J_identification/ipark ==
  dq : Inport  PortDimensions=2
  wt : Inport  Port=2  PortDimensions=1
  Fcn : Fcn  Expr=u[1]*cos(u[3]) - u[2]*sin(u[3])
  Fcn1 : Fcn  Expr=u[1]*sin(u[3]) + u[2]*cos(u[3])
  Mux1 : Mux  Inputs=[2 1]
  Mux2 : Mux  Inputs=[2 1]
  alpha : Outport  InitialOutput=[0,0]
  beta : Outport  Port=2  InitialOutput=[0,0]
  wires:
  Fcn1/1 -> beta/1
  Fcn/1 -> alpha/1
  dq/1 -> Mux1/1, Mux2/1
  Mux1/1 -> Fcn/1
  wt/1 -> Mux1/2, Mux2/2
  Mux2/1 -> Fcn1/1

== system fangbo_pll_eso_J_identification/measurement ==
  m : Inport
  Bus Selector : BusSelector  OutputSignals=Rotor speed wm (rad/s),Rotor angle thetam (rad),Electromagnetic torque Te (N*m),Stator current is_a (A),Stator current is_b (A),Stator current is_c (A)
  Mux : Mux  Inputs=3
  Rate Transition{1..4} (4 alike) : RateTransition  OutPortSampleTime=1e-4
  i : Gain  Gain=30/pi
  i1 : Gain  Gain=Pn
  n : Outport
  thee : Outport  Port=2
  Te : Outport  Port=3
  iabc : Outport  Port=4
  wires:
  m/1 -> Bus Selector/1
  Bus Selector/6 -> Mux/3  "<Stator current is_c (A)>"
  Bus Selector/4 -> Mux/1  "<Stator current is_a (A)>"
  Bus Selector/3 -> Rate Transition3/1  "<Electromagnetic torque Te (N*m)>"
  Bus Selector/5 -> Mux/2  "<Stator current is_b (A)>"
  i/1 -> Rate Transition1/1
  Mux/1 -> Rate Transition4/1
  Bus Selector/1 -> i/1  "<Rotor speed wm (rad/s)>"
  Bus Selector/2 -> i1/1  "<Rotor angle thetam (rad)>"
  i1/1 -> Rate Transition2/1
  Rate Transition1/1 -> n/1
  Rate Transition2/1 -> thee/1
  Rate Transition3/1 -> Te/1
  Rate Transition4/1 -> iabc/1

== system fangbo_pll_eso_J_identification/transform1 ==
  Is : Inport
  wt : Inport  Port=2
  Alpha-Beta-Zero to dq0 : powerlib_meascontrol/Transformations/Alpha-Beta-Zero to dq0  Alignment=Aligned with phase A axis
      settings: SourceProductName=Simscape Electrical
  Demux : Demux  Outputs=3
  Demux1 : Demux  Outputs=3
  Mux2 : Mux  Inputs=3
  Terminator1 : Terminator
  abc to Alpha-Beta-Zero : powerlib_meascontrol/Transformations/abc to Alpha-Beta-Zero
      settings: SourceProductName=Simscape Electrical
  iα : Outport
  iβ : Outport  Port=2
  id : Outport  Port=3
  iq : Outport  Port=4
  wires:
  wt/1 -> Alpha-Beta-Zero to dq0/2
  Demux/3 -> Mux2/3
  Is/1 -> abc to Alpha-Beta-Zero/1
  Demux1/2 -> iq/1  "iq"
  Demux1/1 -> id/1  "id"
  Mux2/1 -> Alpha-Beta-Zero to dq0/1
  abc to Alpha-Beta-Zero/1 -> Demux/1
  Alpha-Beta-Zero to dq0/1 -> Demux1/1  "idq"
  Demux1/3 -> Terminator1/1
  Demux/1 -> Mux2/1, iα/1
  Demux/2 -> Mux2/2, iβ/1

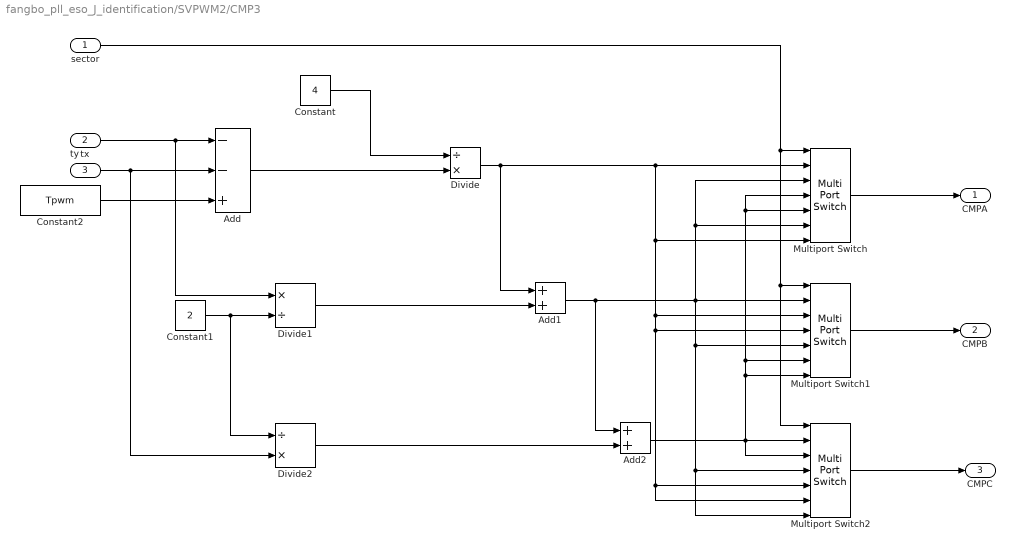
== system fangbo_pll_eso_J_identification/SVPWM2/CMP3 ==
  sector : Inport
  tx : Inport  Port=2
  ty : Inport  Port=3
  Add : Sum  Inputs=--+
  Add1 : Sum
  Add2 : Sum
  Constant : Constant  Value=4
  Constant1 : Constant  Value=2
  Constant2 : Constant  Value=Tpwm
  Divide : Product  Inputs=/*
  Divide1 : Product  Inputs=*/
  Divide2 : Product  Inputs=/*
  Multiport Switch : MultiPortSwitch  Inputs=6
  Multiport Switch1 : MultiPortSwitch  Inputs=6
  Multiport Switch2 : MultiPortSwitch  Inputs=6
  CMPA : Outport
  CMPB : Outport  Port=2
  CMPC : Outport  Port=3
  wires:
  tx/1 -> Add/1, Divide1/1
  ty/1 -> Add/2, Divide2/2
  Constant2/1 -> Add/3
  sector/1 -> Multiport Switch2/1, Multiport Switch1/1, Multiport Switch/1
  Multiport Switch/1 -> CMPA/1
  Add2/1 -> Multiport Switch/4, Multiport Switch/5, Multiport Switch1/6, Multiport Switch1/7, Multiport Switch2/2, Multiport Switch2/3
  Divide2/1 -> Add2/2
  Add1/1 -> Add2/1, Multiport Switch/3, Multiport Switch/6, Multiport Switch1/2, Multiport Switch1/5, Multiport Switch2/4, Multiport Switch2/7
  Divide1/1 -> Add1/2
  Divide/1 -> Add1/1, Multiport Switch/2, Multiport Switch/7, Multiport Switch1/3, Multiport Switch1/4, Multiport Switch2/5, Multiport Switch2/6
  Constant1/1 -> Divide1/2, Divide2/1
  Add/1 -> Divide/2
  Constant/1 -> Divide/1
  Multiport Switch1/1 -> CMPB/1
  Multiport Switch2/1 -> CMPC/1

== system fangbo_pll_eso_J_identification/SVPWM2/PWMlixiang ==
  CMP1 : Inport
  CMP2 : Inport  Port=2
  CMP3 : Inport  Port=3
  Bus Creator : BusCreator  Inputs=6
  Logical Operator : Logic  Operator=NOT  Inputs=1  AllPortsSameDT=off  OutDataTypeStr=boolean
  Logical Operator1 : Logic  Operator=NOT  Inputs=1  AllPortsSameDT=off  OutDataTypeStr=boolean
  Logical Operator2 : Logic  Operator=NOT  Inputs=1  AllPortsSameDT=off  OutDataTypeStr=boolean
  Relational Operator : RelationalOperator  OutDataTypeStr=boolean  RndMeth=Nearest
  Relational Operator1 : RelationalOperator  OutDataTypeStr=boolean  RndMeth=Nearest
  Relational Operator2 : RelationalOperator  OutDataTypeStr=boolean  RndMeth=Nearest
  Scope1 : Scope
  carrier : simulink/Sources/Repeating Sequence  rep_seq_t=[0 Tpwm/2 Tpwm]  rep_seq_y=[0 Tpwm/2 0]
  PWM : Outport
  wires:
  Logical Operator2/1 -> Bus Creator/6
  Relational Operator2/1 -> Bus Creator/5, Logical Operator2/1
  Logical Operator1/1 -> Bus Creator/4
  Relational Operator1/1 -> Bus Creator/3, Logical Operator1/1
  Logical Operator/1 -> Bus Creator/2
  Relational Operator/1 -> Bus Creator/1, Scope1/1, Logical Operator/1
  CMP3/1 -> Relational Operator2/2
  CMP2/1 -> Relational Operator1/2
  Bus Creator/1 -> PWM/1
  CMP1/1 -> Relational Operator/2
  carrier/1 -> Relational Operator2/1, Relational Operator1/1, Relational Operator/1

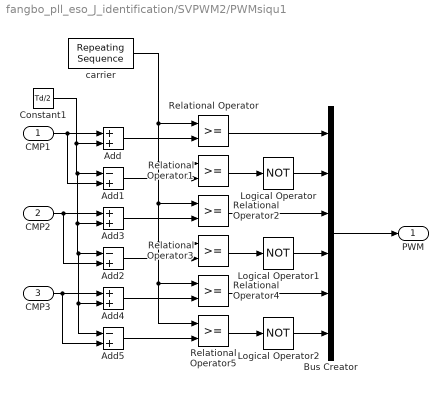
== system fangbo_pll_eso_J_identification/SVPWM2/PWMsiqu1 ==
  CMP1 : Inport
  CMP2 : Inport  Port=2
  CMP3 : Inport  Port=3
  Add : Sum
  Add1 : Sum  Inputs=-+
  Add2 : Sum  Inputs=-+
  Add3 : Sum
  Add4 : Sum
  Add5 : Sum  Inputs=-+
  Bus Creator : BusCreator  Inputs=6
  Constant1 : Constant  Value=Td/2
  Logical Operator : Logic  Operator=NOT  Inputs=1  AllPortsSameDT=off  OutDataTypeStr=boolean
  Logical Operator1 : Logic  Operator=NOT  Inputs=1  AllPortsSameDT=off  OutDataTypeStr=boolean
  Logical Operator2 : Logic  Operator=NOT  Inputs=1  AllPortsSameDT=off  OutDataTypeStr=boolean
  Relational Operator{,1..5} (6 alike) : RelationalOperator  OutDataTypeStr=boolean  RndMeth=Nearest
  carrier : simulink/Sources/Repeating Sequence  rep_seq_t=[0 Tpwm/2 Tpwm]  rep_seq_y=[0 Tpwm/2 0]
  PWM : Outport
  wires:
  Logical Operator2/1 -> Bus Creator/6
  Relational Operator4/1 -> Bus Creator/5
  Logical Operator1/1 -> Bus Creator/4
  Relational Operator2/1 -> Bus Creator/3
  Logical Operator/1 -> Bus Creator/2
  Relational Operator/1 -> Bus Creator/1
  Add4/1 -> Relational Operator4/2
  Add3/1 -> Relational Operator2/2
  Bus Creator/1 -> PWM/1
  Add/1 -> Relational Operator/2
  carrier/1 -> Relational Operator1/1, Relational Operator2/1, Relational Operator3/1, Relational Operator5/1, Relational Operator4/1, Relational Operator/1
  CMP1/1 -> Add1/2, Add/1
  Constant1/1 -> Add3/2, Add5/1, Add4/2, Add2/1, Add1/1, Add/2
  Add1/1 -> Relational Operator1/2
  Relational Operator1/1 -> Logical Operator/1
  Relational Operator5/1 -> Logical Operator2/1
  Add2/1 -> Relational Operator3/2
  Add5/1 -> Relational Operator5/2
  CMP3/1 -> Add5/2, Add4/1
  CMP2/1 -> Add2/2, Add3/1
  Relational Operator3/1 -> Logical Operator1/1

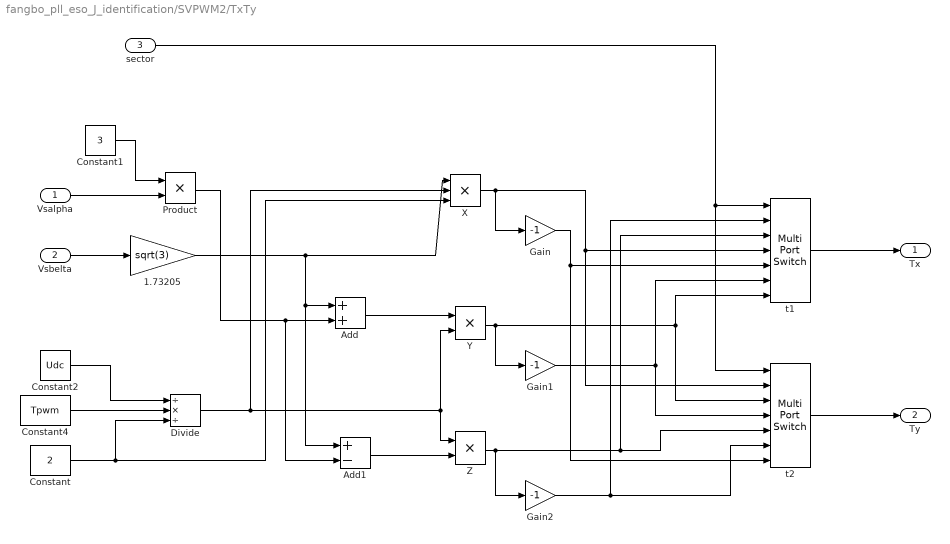
== system fangbo_pll_eso_J_identification/SVPWM2/TxTy ==
  Vsalpha : Inport
  Vsbelta : Inport  Port=2
  sector : Inport  Port=3
  1.73205 : Gain  Gain=sqrt(3)
  Add : Sum
  Add1 : Sum  Inputs=+-
  Constant : Constant  Value=2
  Constant1 : Constant  Value=3
  Constant2 : Constant  Value=Udc
  Constant4 : Constant  Value=Tpwm
  Divide : Product  Inputs=/*/
  Gain : Gain  Gain=-1
  Gain1 : Gain  Gain=-1
  Gain2 : Gain  Gain=-1
  Product : Product  RndMeth=Zero
  X : Product  Inputs=3  RndMeth=Zero
  Y : Product  RndMeth=Zero
  Z : Product  RndMeth=Zero
  t1 : MultiPortSwitch  Inputs=6
  t2 : MultiPortSwitch  Inputs=6
  Tx : Outport
  Ty : Outport  Port=2
  wires:
  Constant4/1 -> Divide/2
  Constant2/1 -> Divide/1
  Constant/1 -> Divide/3, X/3
  Vsalpha/1 -> Product/2
  Constant1/1 -> Product/1
  Vsbelta/1 -> 1.73205/1
  1.73205/1 -> X/1, Add/1, Add1/1
  Divide/1 -> X/2, Y/2, Z/1
  Product/1 -> Add/2, Add1/2
  Add/1 -> Y/1
  Add1/1 -> Z/2
  X/1 -> Gain/1, t1/4, t2/2
  Y/1 -> Gain1/1, t1/7, t2/3
  Z/1 -> Gain2/1, t1/3, t2/5
  sector/1 -> t2/1, t1/1
  Gain2/1 -> t1/2, t2/6
  Gain/1 -> t1/5, t2/7
  Gain1/1 -> t1/6, t2/4
  t1/1 -> Tx/1
  t2/1 -> Ty/1

== system fangbo_pll_eso_J_identification/SVPWM2/sector ==
  Ualpha : Inport
  Ubeta : Inport  Port=2
  Add : Sum  Inputs=+-
  Add1 : Sum  Inputs=--
  Add2 : Sum  Inputs=+++
  Compare To Zero{,1..3} (4 alike) : simulink/Logic and Bit Operations/Compare To Zero  relop=>  OutDataTypeStr=uint8
  Constant : Constant  Value=1.73205
  Gain : Gain  Gain=4
  Gain1 : Gain  Gain=2
  Lookup Table : Lookup  InputValues=[1,2,3,4,5,6]  Table=[2,6,1,4,3,5]  LookUpMeth=Use Input Below
  Product : Product  RndMeth=Zero
  sector : Outport
  wires:
  Ubeta/1 -> Add/2, Add1/2, Compare To Zero/1
  Ualpha/1 -> Product/2
  Lookup Table/1 -> sector/1
  Add2/1 -> Lookup Table/1
  Compare To Zero1/1 -> Add2/3
  Gain/1 -> Add2/1
  Gain1/1 -> Add2/2
  Compare To Zero3/1 -> Gain/1
  Add1/1 -> Compare To Zero3/1
  Add/1 -> Compare To Zero2/1
  Compare To Zero/1 -> Compare To Zero1/1
  Product/1 -> Add1/1, Add/1
  Constant/1 -> Product/1
  Compare To Zero2/1 -> Gain1/1

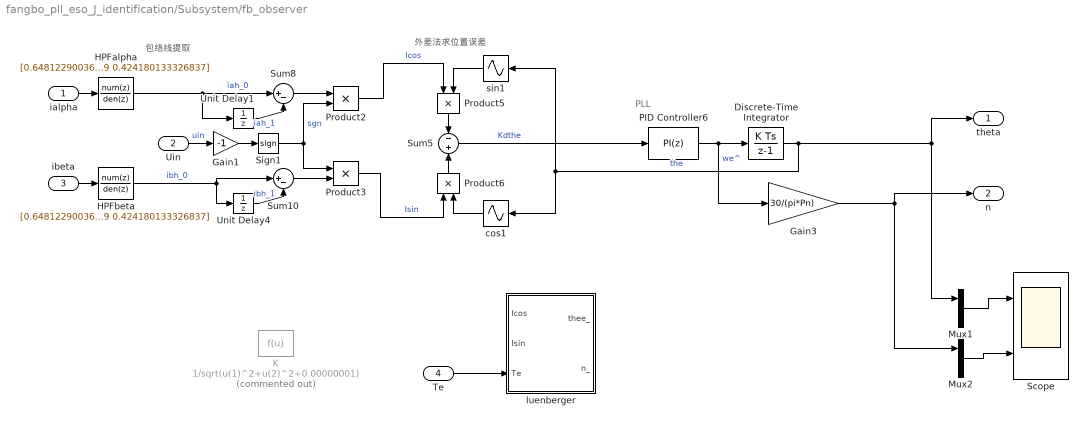
== system fangbo_pll_eso_J_identification/Subsystem/fb_observer ==
  note: PLL
  note: 外差法求位置误差
  note: 包络线提取
  ialpha : Inport
  Uin : Inport  Port=2
  ibeta : Inport  Port=3
  Te : Inport  Port=4
  Discrete-Time Integrator : DiscreteIntegrator  SampleTime=Tpwm  ICPrevOutput=DiscIntNeverNeededParam  ICPrevScaledInput=DiscIntNeverNeededParam
  Gain1 : Gain  Gain=-1
  Gain3 : Gain  Gain=30/(pi*Pn)
  HPFalpha : DiscreteTransferFcn  Numerator=[0.648122900364569 -1.296245800729138 0.648122900364569]  Denominator=[1 -1.168311468131439 0.424180133326837]  SampleTime=Tpwm
  HPFbeta : DiscreteTransferFcn  Numerator=[0.648122900364569 -1.296245800729138 0.648122900364569]  Denominator=[1 -1.168311468131439 0.424180133326837]  SampleTime=Tpwm
  K : Fcn  Commented=on  Expr=1/sqrt(u(1)^2+u(2)^2+0.00000001)
  Mux1 : Mux  Inputs=2
  Mux2 : Mux  Inputs=2
  PID Controller6 : simulink/Continuous/PID Controller  Controller=PI  Form=Ideal  TimeDomain=Discrete-time  SampleTime=Tpwm  IntegratorMethod=Forward Euler  FilterMethod=Forward Euler  ControllerParametersSource=internal  P=5000  I=500  D=0  UseFilter=on  N=100  TunerSelectOption=Transfer Function Based (PID Tuner App)  InitialConditionSource=internal  InitialConditionForIntegrator=0  InitialConditionForFilter=0  DifferentiatorICPrevScaledInput=0  ExternalReset=none  TrackingMode=off  Kt=1  LimitOutput=off  UpperSaturationLimit=inf  LowerSaturationLimit=-inf  LinearizeAsGain=on  AntiWindupMode=none  Kb=1  POutMin=[]  POutMax=[]  IOutMin=[]  IOutMax=[]  DOutMin=[]  DOutMax=[]  NOutMin=[]  NOutMax=[]  SumOutMin=[]  SumOutMax=[]  SaturationOutMin=[]  SaturationOutMax=[]  PParamMin=[]  PParamMax=[]  IParamMin=[]  IParamMax=[]  DParamMin=[]  DParamMax=[]  NParamMin=[]  NParamMax=[]  KbParamMin=[]  KbParamMax=[]  KtParamMin=[]  KtParamMax=[]  KbOutMin=[]  KbOutMax=[]  KtOutMin=[]  KtOutMax=[]  IntegratorOutMin=[]  IntegratorOutMax=[]  FilterOutMin=[]  FilterOutMax=[]  SumI1OutMin=[]  SumI1OutMax=[]  SumI2OutMin=[]  SumI2OutMax=[]  SumI3OutMin=[]  SumI3OutMax=[]  SumI4OutMin=[]  SumI4OutMax=[]  SumDOutMin=[]  SumDOutMax=[]  DifferentiatorOutMin=[]  DifferentiatorOutMax=[]  FilterDiffOutCoefMin=[]  FilterDiffOutCoefMax=[]  ReciprocalOutMin=[]  ReciprocalOutMax=[]  SumDenOutMin=[]  SumDenOutMax=[]  SumNumOutMin=[]  SumNumOutMax=[]  DivideOutMin=[]  DivideOutMax=[]  IntegratorContinuousStateAttributes=''  IntegratorStateMustResolveToSignalObject=off  IntegratorRTWStateStorageClass=Auto  FilterContinuousStateAttributes=''  FilterStateMustResolveToSignalObject=off  FilterRTWStateStorageClass=Auto  ParallelPVariant=Passthrough  IdealPVariant=InternalParameters  IVariant=InternalParameters  DVariant=Disabled  IntegratorVariant=Discrete  SatVariant=Disabled  AWVariant=Passthrough  PCopyVariant=Disabled  TRVariant=Disabled  FdbkBlocksVariant=Forward  IdealPFdbkVariant=Disabled  SatFdbkVariant=Disabled  DerivativeFilterVariant=Disabled  NVariant=Disabled  NCopyVariant=Disabled_SignalSpec  FilterICVariant=Disabled  IntegratorICVariant=InternalICs  ExternalResetVariant=Disabled  TRSumVariant=Passthrough  SumFdbkVariant=Disabled  SumVariant=Sum_PI
  Product{2..3,5..6} (4 alike) : Product
  Scope : Scope  NumInputPorts=2
  Sign1 : Signum
  Sum10 : Sum  Inputs=|+-
  Sum5 : Sum  Inputs=-|+
  Sum8 : Sum  Inputs=|+-
  Unit Delay1 : UnitDelay  SampleTime=Tpwm
  Unit Delay4 : UnitDelay  SampleTime=Tpwm
  cos1 : Sin  TimeSource=Use external signal  Phase=pi/2  SampleTime=0
  luenberger : Subsystem
  sin1 : Sin  TimeSource=Use external signal  SampleTime=0
  theta : Outport
  n : Outport  Port=2
  wires:
  cos1/1 -> Product6/2
  HPFbeta/1 -> Sum10/1, Unit Delay4/1  "ibh_0"
  Sign1/1 -> Product2/2, Product3/1  "sgn"
  Sum5/1 -> PID Controller6/1  "Kdthe"
  PID Controller6/1 -> Discrete-Time Integrator/1, Gain3/1  "we^"
  Sum10/1 -> Product3/2
  Sum8/1 -> Product2/1
  Discrete-Time Integrator/1 -> sin1/1, cos1/1, theta/1, Mux1/1  "the"
  Gain3/1 -> n/1, Mux2/1
  Product2/1 -> Product5/1  "Icos"
  Gain1/1 -> Sign1/1
  Product3/1 -> Product6/1  "Isin"
  Product5/1 -> Sum5/1
  Unit Delay4/1 -> Sum10/2  "ibh_1"
  Product6/1 -> Sum5/2
  sin1/1 -> Product5/2
  Uin/1 -> Gain1/1  "uin"
  HPFalpha/1 -> Unit Delay1/1, Sum8/1  "iah_0"
  Unit Delay1/1 -> Sum8/2  "iah_1"
  ialpha/1 -> HPFalpha/1
  ibeta/1 -> HPFbeta/1
  Mux1/1 -> Scope/1
  Mux2/1 -> Scope/2
  Te/1 -> luenberger/3(Te)

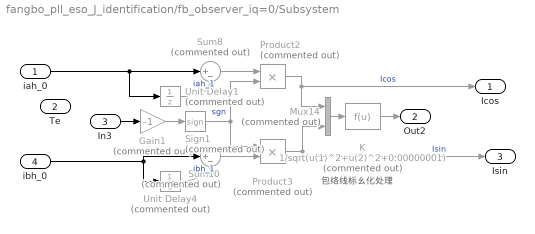
== system fangbo_pll_eso_J_identification/fb_observer_iq=0/Subsystem ==
  note: 包络线标幺化处理
  iah_0 : Inport
  Te : Inport  Port=2
  In3 : Inport  Port=3
  ibh_0 : Inport  Port=4
  Gain1 : Gain  Commented=on  Gain=-1
  K : Fcn  Commented=on  Expr=1/sqrt(u(1)^2+u(2)^2+0.00000001)
  Mux14 : Mux  Commented=on  Inputs=2
  Product2 : Product  Commented=on
  Product3 : Product  Commented=on
  Sign1 : Signum  Commented=on
  Sum10 : Sum  Commented=on  Inputs=|+-
  Sum8 : Sum  Commented=on  Inputs=|+-
  Unit Delay1 : UnitDelay  Commented=on  SampleTime=Tpwm
  Unit Delay4 : UnitDelay  Commented=on  SampleTime=Tpwm
  Icos : Outport
  Out2 : Outport  Port=2
  Isin : Outport  Port=3
  wires:
  Mux14/1 -> K/1
  Product2/1 -> Icos/1, Mux14/1  "Icos"
  Unit Delay4/1 -> Sum10/2  "ibh_1"
  Product3/1 -> Isin/1, Mux14/2  "Isin"
  iah_0/1 -> Sum8/1, Unit Delay1/1
  Sum8/1 -> Product2/1
  Unit Delay1/1 -> Sum8/2  "iah_1"
  Sum10/1 -> Product3/2
  Gain1/1 -> Sign1/1
  Sign1/1 -> Product3/1, Product2/2  "sgn"
  ibh_0/1 -> Unit Delay4/1, Sum10/1
  K/1 -> Out2/1
  In3/1 -> Gain1/1

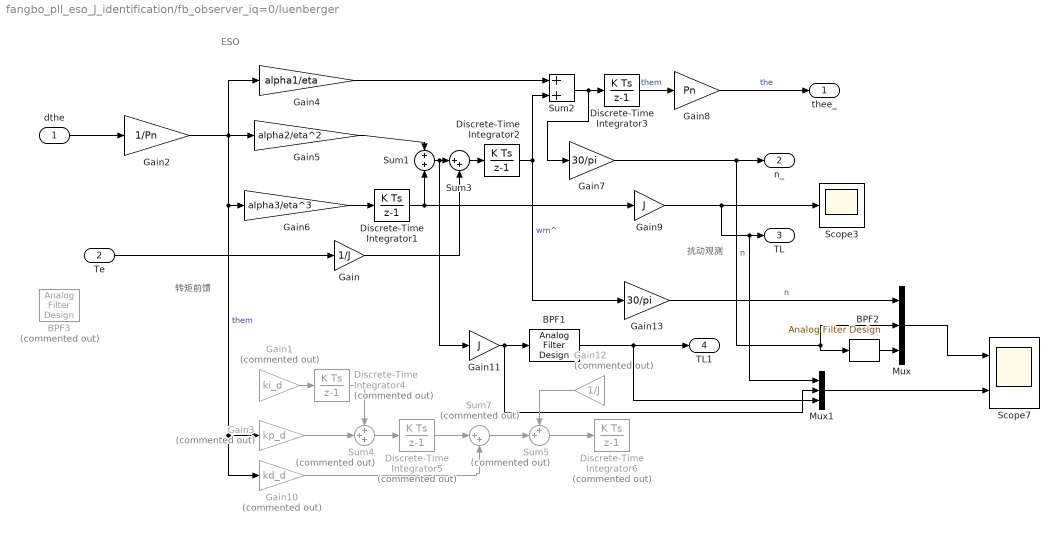
== system fangbo_pll_eso_J_identification/fb_observer_iq=0/luenberger ==
  note: 转矩前馈
  note: ESO
  note: 扰动观测
  dthe : Inport
  Te : Inport  Port=2
  BPF1 : dsparch4/Analog Filter Design  method=Butterworth  filttype=Lowpass  N=2  Wlo=100*2*pi  Whi=(fin+200)*2*pi  Rp=2  Rs=40
  BPF2 : dsparch4/Analog Filter Design  method=Butterworth  filttype=Lowpass  N=1  Wlo=wcon  Whi=(fin+200)*2*pi  Rp=2  Rs=40
  BPF3 : dsparch4/Analog Filter Design  Commented=on  method=Butterworth  filttype=Lowpass  N=1  Wlo=100*2*pi  Whi=(fin+200)*2*pi  Rp=2  Rs=40
  Discrete-Time Integrator1 : DiscreteIntegrator  SampleTime=Tpwm  ICPrevOutput=DiscIntNeverNeededParam  ICPrevScaledInput=DiscIntNeverNeededParam
  Discrete-Time Integrator2 : DiscreteIntegrator  SampleTime=Tpwm  ICPrevOutput=DiscIntNeverNeededParam  ICPrevScaledInput=DiscIntNeverNeededParam
  Discrete-Time Integrator3 : DiscreteIntegrator  SampleTime=Tpwm  ICPrevOutput=DiscIntNeverNeededParam  ICPrevScaledInput=DiscIntNeverNeededParam
  Discrete-Time Integrator4 : DiscreteIntegrator  Commented=on  SampleTime=Tpwm  ICPrevOutput=DiscIntNeverNeededParam  ICPrevScaledInput=DiscIntNeverNeededParam
  Discrete-Time Integrator5 : DiscreteIntegrator  Commented=on  SampleTime=Tpwm  ICPrevOutput=DiscIntNeverNeededParam  ICPrevScaledInput=DiscIntNeverNeededParam
  Discrete-Time Integrator6 : DiscreteIntegrator  Commented=on  SampleTime=Tpwm  ICPrevOutput=DiscIntNeverNeededParam  ICPrevScaledInput=DiscIntNeverNeededParam
  Gain : Gain  Gain=1/J
  Gain1 : Gain  Commented=on  Gain=ki_d
  Gain10 : Gain  Commented=on  Gain=kd_d
  Gain11 : Gain  Gain=J
  Gain12 : Gain  Commented=on  Gain=1/J
  Gain13 : Gain  Gain=30/pi
  Gain2 : Gain  Gain=1/Pn
  Gain3 : Gain  Commented=on  Gain=kp_d
  Gain4 : Gain  Gain=alpha1/eta
  Gain5 : Gain  Gain=alpha2/eta^2
  Gain6 : Gain  Gain=alpha3/eta^3
  Gain7 : Gain  Gain=30/pi
  Gain8 : Gain  Gain=Pn
  Gain9 : Gain  Gain=J
  Mux : Mux  Inputs=3
  Mux1 : Mux  Inputs=3
  Scope3 : Scope
  Scope7 : Scope  NumInputPorts=2
  Sum1 : Sum  Inputs=+|+
  Sum2 : Sum
  Sum3 : Sum  Inputs=|++
  Sum4 : Sum  Commented=on  Inputs=+++
  Sum5 : Sum  Commented=on  Inputs=++|
  Sum7 : Sum  Commented=on  Inputs=|++
  thee_ : Outport
  n_ : Outport  Port=2
  TL : Outport  Port=3
  TL1 : Outport  Port=4
  wires:
  Gain7/1 -> BPF2/1, Mux/2, n_/1  "n"
  Gain9/1 -> Mux1/1, TL/1, Scope3/1
  Gain2/1 -> Gain4/1, Gain5/1, Gain10/1, Gain3/1, Gain6/1  "them"
  Gain5/1 -> Sum1/1
  Te/1 -> Gain/1
  Gain6/1 -> Discrete-Time Integrator1/1
  Discrete-Time Integrator1/1 -> Sum1/2, Gain9/1
  Sum2/1 -> Gain7/1, Discrete-Time Integrator3/1
  Sum1/1 -> Gain11/1, Sum3/1
  Gain/1 -> Sum3/2
  Gain4/1 -> Sum2/1
  Discrete-Time Integrator2/1 -> Gain13/1, Sum2/2  "wm^"
  Gain8/1 -> thee_/1  "the"
  Discrete-Time Integrator3/1 -> Gain8/1  "them"
  dthe/1 -> Gain2/1
  Gain1/1 -> Discrete-Time Integrator4/1
  Gain3/1 -> Sum4/2
  Gain10/1 -> Sum7/2
  Sum7/1 -> Sum5/2
  Gain11/1 -> Mux1/2, BPF1/1
  ? -> Gain12/1
  Gain12/1 -> Sum5/1
  Sum5/1 -> Discrete-Time Integrator6/1
  Mux/1 -> Scope7/1
  Mux1/1 -> Scope7/2
  Discrete-Time Integrator4/1 -> Sum4/1
  Discrete-Time Integrator5/1 -> Sum7/1
  Sum4/1 -> Discrete-Time Integrator5/1
  Sum3/1 -> Discrete-Time Integrator2/1
  BPF1/1 -> Mux1/3, TL1/1
  Gain13/1 -> Mux/1  "n"
  BPF2/1 -> Mux/3
